simulink model "Solar_Seguidor_V2"  (R2021b)
settings: Solver=ode1  StartTime=0.0  StopTime=10  FixedStep=25e-6  RelTol=1e-3
PostLoadFcn:
  | %clc; clear all; close all;
  | %%%%%%%%%%%%%%%%%%%%%%%%%%%%%%%%%%%%%%%%%%%%%%%%
  | %%%%%%%%% Solar seguidor de rede %%%%%%%%%%
  | %%%%%%%%%%%%%%%%%%%%%%%%%%%%%%%%%%%%%%%%%%%%%%%%
  | %%%% Nominal Parameters %%%%
  | Pnom = 16e3;                                         % Potencia Nominal
  | Vnom_rms = 210;                                    % V linha rms
  | Vnom_peak = sqrt(2/3)*Vnom_rms;                     % V fase pico
  | FP_min = 1;                                       % Para suporte de reativo
  | Snom = Pnom/FP_min;                                 % Potencia aparente
  | Irms = Pnom/(sqrt(3)*Vnom_rms);                     % Ig rms
  | Inom_peak = Irms*sqrt(2);                           % Ig pico
  | Zbase = Vnom_peak/Inom_peak;                        % Impedancia Base
  | f = 60;                                             % Freq nominal
  | wnom = 2*pi*60;                                     % Freq Ang. nominal
  | m = 0.805;                                            % Indice mod nominal
  | Vdc = 2*(Vnom_peak/m);                              % Vcc
  | Vdc_2 = Vdc/2;                                      % Metade Vcc
  | Kconv = Zbase;                                      % Ganho conversor
  | %%%% Transformer %%%%
  | S_trafo = 250e3;                                      % transformer apparent power
  | Vrms_high = 400;                                   % transformer secondary voltage - Wye connection
  | Vrms_low = 210;                                   % transformer primary voltage - Delta connection
  | N = Vrms_high/Vrms_low;                             % transformation relationship
  | X_pu_trafo = 0.03;                                 % transformer p.u. reactance
  | Zb_trafo_high = ((Vrms_high)^2)/S_trafo;            % secondary base impedance
  | Zb_trafo = ((Vnom_rms)^2)/S_trafo;                  % primary base impedance
  | L_trafo = (X_pu_trafo*Zb_trafo)/wnom;               % primary inductance
  | %%%% LCL Filter Project %%%%
  | fsw = 105*60;%105*60;                                         % switching frequency
  | ripple = 0.05;                                       % current ripple
  | L1 = Vdc/(6*ripple*Inom_peak*fsw);                  % inductor L1
  |  RL1 = 0.005;                                        % L1 resistance
  |  Cbase = 1/(wnom*Kconv);                             % base capacitance
  |  Cf = 0.05*Cbase;                                    % filter capacitor
  | % Calculo do filtro
  | Sbase = 16e3;
  | %Sbase = 200e3*1.12;
  | V_LL = 210;
  | V_LG = 210/sqrt(3);
  | Vbase = V_LG*sqrt(2);
  | Ibase = (Sbase*sqrt(2))/(V_LG*3)*sqrt(3/2);
  | Zbase = (V_LL^2)/Sbase;
  | Rbase = Zbase;
  | Xbase = Zbase;
  | Lbase = Xbase/(2*pi*60);
  | Cbase = 1/(Xbase*2*pi*60);
  | w = 2*pi*60;
  | Q = 70;
  | Lf = 0.15*Lbase;
  | Cf = 0.05*Cbase;
  | fc = 1/(2*pi*sqrt(Lf*Cf));
  | R = (w*Lf)/Q;
  | Lf = L1;
  | R = RL1;
  | ka=0.2;                                             % attenuation factor
  | L2 = (sqrt(1/(ka^2))+1)/(Cf*((2*pi*fsw)^2));        % inductor L2
  | RL2 = 0.005;                                        % L2 resistance
  | w_res = sqrt((L1+L2+L_trafo)/(L1*L2*Cf));           % resonant angular frequency
  | f_res = w_res/(2*pi);                               % resonant frequency
  | ... (+31 lines)
InitFcn:
  | %clc; clear all; close all;
  | %%%%%%%%%%%%%%%%%%%%%%%%%%%%%%%%%%%%%%%%%%%%%%%%
  | %%%%%%%%% Solar seguidor de rede %%%%%%%%%%
  | %%%%%%%%%%%%%%%%%%%%%%%%%%%%%%%%%%%%%%%%%%%%%%%%
  | %%%% Nominal Parameters %%%%
  | Pnom = 16e3;                                         % Potencia Nominal
  | Vnom_rms = 210;                                    % V linha rms
  | Vnom_peak = sqrt(2/3)*Vnom_rms;                     % V fase pico
  | FP_min = 1;                                       % Para suporte de reativo
  | Snom = Pnom/FP_min;                                 % Potencia aparente
  | Irms = Pnom/(sqrt(3)*Vnom_rms);                     % Ig rms
  | Inom_peak = Irms*sqrt(2);                           % Ig pico
  | Zbase = Vnom_peak/Inom_peak;                        % Impedancia Base
  | f = 60;                                             % Freq nominal
  | wnom = 2*pi*60;                                     % Freq Ang. nominal
  | m = 0.805;                                            % Indice mod nominal
  | Vdc = 2*(Vnom_peak/m);                              % Vcc
  | Vdc_2 = Vdc/2;                                      % Metade Vcc
  | Kconv = Zbase;                                      % Ganho conversor
  | %%%% Transformer %%%%
  | S_trafo = 250e3;                                      % transformer apparent power
  | Vrms_high = 400;                                   % transformer secondary voltage - Wye connection
  | Vrms_low = 210;                                   % transformer primary voltage - Delta connection
  | N = Vrms_high/Vrms_low;                             % transformation relationship
  | X_pu_trafo = 0.03;                                 % transformer p.u. reactance
  | Zb_trafo_high = ((Vrms_high)^2)/S_trafo;            % secondary base impedance
  | Zb_trafo = ((Vnom_rms)^2)/S_trafo;                  % primary base impedance
  | L_trafo = (X_pu_trafo*Zb_trafo)/wnom;               % primary inductance
  | %%%% LCL Filter Project %%%%
  | fsw = 105*60;%105*60;                                         % switching frequency
  | ripple = 0.05;                                       % current ripple
  | L1 = Vdc/(6*ripple*Inom_peak*fsw);                  % inductor L1
  |  RL1 = 0.005;                                        % L1 resistance
  |  Cbase = 1/(wnom*Kconv);                             % base capacitance
  |  Cf = 0.05*Cbase;                                    % filter capacitor
  | % Calculo do filtro
  | Sbase = 16e3;
  | %Sbase = 200e3*1.12;
  | V_LL = 210;
  | V_LG = 210/sqrt(3);
  | Vbase = V_LG*sqrt(2);
  | Ibase = (Sbase*sqrt(2))/(V_LG*3)*sqrt(3/2);
  | Zbase = (V_LL^2)/Sbase;
  | Rbase = Zbase;
  | Xbase = Zbase;
  | Lbase = Xbase/(2*pi*60);
  | Cbase = 1/(Xbase*2*pi*60);
  | w = 2*pi*60;
  | Q = 70;
  | Lf = 0.15*Lbase;
  | Cf = 0.05*Cbase;
  | fc = 1/(2*pi*sqrt(Lf*Cf));
  | R = (w*Lf)/Q;
  | Lf = L1;
  | R = RL1;
  | ka=0.2;                                             % attenuation factor
  | L2 = (sqrt(1/(ka^2))+1)/(Cf*((2*pi*fsw)^2));        % inductor L2
  | RL2 = 0.005;                                        % L2 resistance
  | w_res = sqrt((L1+L2+L_trafo)/(L1*L2*Cf));           % resonant angular frequency
  | f_res = w_res/(2*pi);                               % resonant frequency
  | ... (+31 lines)
undefined symbols (not defined in the file): D1, Delta, DERS_models, DiscIntNeverNeededParam, eHS, I, Ia_PV, Ib_PV, Ic_PV, Left, parameter_set_id, ph, PV_system, type, V, Va_grid, Vb_grid, Vc_grid
libraries: powerlib_meascontrol x17, rtlab x14, spsThreePhaseSeriesRLCBranchLib x9, spsCurrentMeasurementLib x9, artemis x7, spsThreePhaseVIMeasurementLib x6, slpidlib x6, rteventslib x6, spsabctodq0Lib x4, spsThreePhaseTransformerTwoWindingsLib x3, simulink x3, spsPVArrayLib x3
(part 2 of 4)

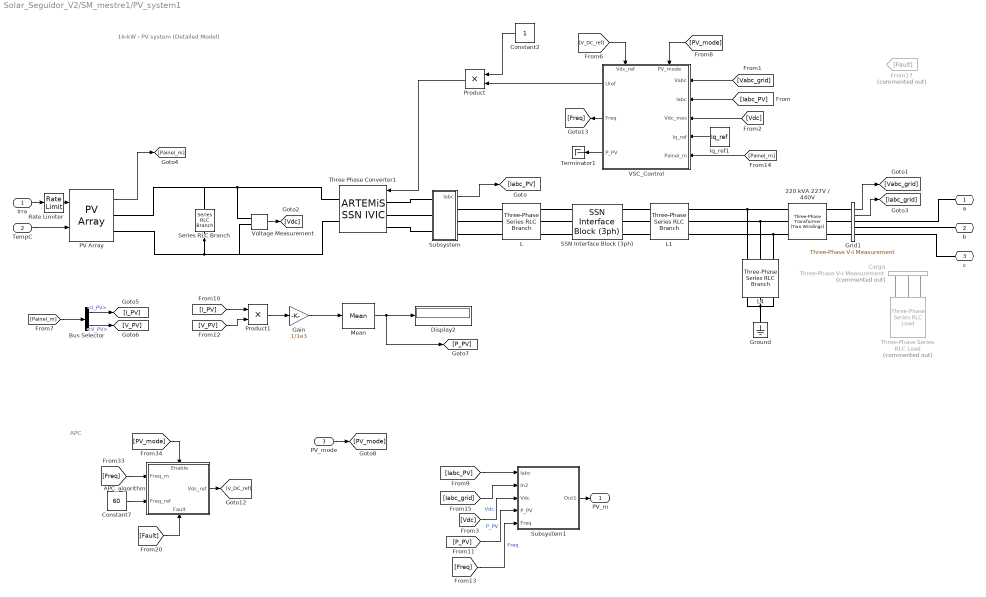
== system Solar_Seguidor_V2/SM_mestre1/PV_system1 ==
  note: APC
  note: 16-kW - PV system (Detailed Model)
  Irra : Inport
  TempC : Inport  Port=2
  PV_mode : Inport  Port=3
  220 kVA 227V / 440V : spsThreePhaseTransformerTwoWindingsLib/Three-Phase Transformer (Two Windings)  Winding1Connection=Yg  Winding2Connection=Delta (D1)  CoreType=Three single-phase transformers  SetSaturation=off  Hysteresis=off  DataFile='hysteresis'  SetInitialFlux=off  Measurements=None  UNITS=pu  NominalPower=[220e3 , 60 ]  Winding1=[400 , 0.001 , 0.03 ]  Winding2=[210 , 0.001 , 0.03 ]  Rm=500  Lm=500  L0=0.5  Saturation=[ 0,0 ; 0.0024,1.2 ; 1.0,1.52 ]  InitialFluxes=[ 0.8 , -0.8 , 0.7 ]  BreakLoop=off  DiscreteSolver=Trapezoidal iterative  DataType=off  TransfoNumber=0
  APC_algorithm : Subsystem
      settings: PortSchema="{\"entries\":[{\"content\":{\"sides\":[{\"content\":{\"connectorIds\":[\"In1\",\"In2\"]},\"type\":\"ConnectorPlacement.EquallySpacedRectSide\",\"uuid\":\"40656380-5e11-4201-a16e-0974ed2bdfa3\"},{\"content\":{\"connectorIds\":[\"Out1\"],\"side\":\"RIGHT\"},\"type\":\"ConnectorPlacement.EquallySpacedRectSide\",\"uuid\":\"b720f4a2-445d-4911-b95b-a16e7ba2ef90\"},{\"content\":{\"connectorIds\":[\"In3\"],\"side\":\"TOP\"},\"type\":\"ConnectorPlacement.EquallySpacedRectSide\",\"uuid\":\"61735eee-8c6f-4b86-833d-6912c6cea25a\"},{\"content\":{\"connectorIds\":[\"In4\"],\"side\":\"BOTTOM\"},\"type\":\"ConnectorPlacement.EquallySpacedRectSide\",\"uuid\":\"0dbf41d0-9732-4713-8148-d584ab86d8ba\"},{\"content\":{\"connectorIds\":[],\"side\":\"HIDDEN\"},\"type\":\"ConnectorPlacement.EquallySpacedRectSide\",\"uuid\":\"d2c68c6b-be31-4766-a941-11238d66741c\"}]},\"type\":\"ConnectorPlacement.EquallySpacedConnector\",\"uuid\":\"e0287d46-a6c7-46a5-bd63-f4e94fb98690\"}],\"packageUris\":[\"http://schema.mathworks.com/mf0/Connector/R2020b\"],\"version\":\"1.0\"}"
  Bus Selector : BusSelector  OutputSignals=I_PV,V_PV
  Carga : spsThreePhaseVIMeasurementLib/Three-Phase V-I Measurement  Commented=on  VoltageMeasurement=phase-to-ground  SetLabelV=on  LabelV=Vcarga  Vpu=off  VpuLL=off  CurrentMeasurement=yes  SetLabelI=on  LabelI=Icarga  Ipu=off  Pbase=100e6  Vbase=500e3  OutputType=Magnitude  PhasorSimulation=off  PSBequivalent=0
  Constant2 : Constant
  Constant7 : Constant  Value=60
  Display2 : Display
  From17 : From  Commented=on  GotoTag=Fault
  Gain : Gain  Gain=1/1e3
  Grid1 : spsThreePhaseVIMeasurementLib/Three-Phase V-I Measurement  VoltageMeasurement=phase-to-ground  SetLabelV=off  LabelV=Vabc_grid  Vpu=off  VpuLL=off  CurrentMeasurement=yes  SetLabelI=off  LabelI=Iabc_grid  Ipu=off  Pbase=100e6  Vbase=500e3  OutputType=Magnitude  PhasorSimulation=off  PSBequivalent=0
  Ground : spsGroundLib/Ground  LConnTagsString=a
  Iq_ref1 : Constant  Value=Iq_ref
  L : spsThreePhaseSeriesRLCBranchLib/Three-Phase Series RLC Branch  LConnTagsString=A|B|C  RConnTagsString=A|B|C  BranchType=R  Resistance=R  Inductance=500e-6/2  Capacitance=inf  Measurements=None
  L1 : spsThreePhaseSeriesRLCBranchLib/Three-Phase Series RLC Branch  LConnTagsString=A|B|C  RConnTagsString=A|B|C  BranchType=L  Resistance=500e-6*377/50/2  Inductance=Lf  Capacitance=inf  Measurements=None
  L4 : spsThreePhaseSeriesRLCBranchLib/Three-Phase Series RLC Branch  LConnTagsString=A|B|C  RConnTagsString=A|B|C  BranchType=R  Resistance=1e8  Inductance=Lf  Capacitance=Cf  Measurements=None
  Mean : spsMeanLib/Mean  Freq=60  Vinit=0  Ts=0
  PV Array : spsPVArrayLib/PV Array  Npar=5  Nser=14  PlotType=array @ 1000 W/m2 & specified temperatures  S_vec=[ 1000]  Temp_C_vec=[ 25 ]  ModuleName=Trina Solar TSM-240PA05.30  PlotWhenSelected=off  Pm=239.856  Ncell=60  Voc=37.2  Isc=8.37  Vm=30.4  Im=7.89  beta_Voc_pc=-0.35  alpha_Isc_pc=0.06  beta_Voc=-0.1302  alpha_Isc=0.005022  IL=8.3942  I0=1.9964e-10  nI=0.98701  Rsh=355.1808  Rs=0.28785  RobustModel=off  RobustCellTemperature=313.3991  BAL=on  Tc=1e-6  Tfilter=5e-5
      settings: AttributesFormatString=|
      | %<ModuleName>
      | %<Nser>-module string
      | %<Npar> parallel strings
  Product : Product
  Product1 : Product
  Rate Limiter : RateLimiter  RisingSlewLimit=5000  FallingSlewLimit=-5000  SampleTimeMode=inherited  LinearizeAsGain=off
  SSN Interface Block (3ph) : artemis/SSN/Nodal Interface Blocks/SSN Interface Block (3ph)  nb_phase=3  nb_port=2  p1_type=I-type(Left)  p2_type=V-type (Right)  p3_type=V-type(Left)  p4_type=V-type(Left)  p5_type=V-type(Left)  p6_type=V-type(Left)  p7_type=V-type(Left)  p8_type=V-type(Left)  p9_type=V-type(Left)  p10_type=V-type(Left)  p11_type=V-type(Left)  p12_type=V-type(Left)  p13_type=V-type(Left)  p14_type=V-type(Left)  p15_type=V-type(Left)  p16_type=V-type(Left)  I_port_shunt_resistance=1e9
  Series RLC Branch : spsSeriesRLCBranchLib/Series RLC Branch  LConnTagsString=__new0  RConnTagsString=__new0  BranchType=C  Resistance=1  Inductance=1e-3  SetiL0=off  InitialCurrent=0  Capacitance=C_cc_proj  Setx0=on  InitialVoltage=Vdc  Measurements=None
  Subsystem : Subsystem
  Subsystem1 : Subsystem
  Terminator1 : Terminator
  Three Phase Converter1 : ssn_inverter_model/ARTEMiS SSN IVIC  Arms=3  SnubberResistance=800  SnubberCapacitance=inf  Device=IGBT / Diodes  Ron=Ron  Lon=0  ForwardVoltages=[0.001 0.001]  ForwardVoltage=0  GTOparameters=[ 10e-6 , 20e-6 ]  IGBTparameters=[ 1e-6 , 2e-6 ]*0  Measurements=None  Measurements_2=None  converterType=Rectifier
  Three-Phase Series RLC Load : spsThreePhaseSeriesRLCLoadLib/Three-Phase Series RLC Load  Commented=on  LConnTagsString=A|B|C  Configuration=Y (grounded)  NominalVoltage=227  Vabc=[1e3 1e3 1e3]  Vabcp=[1e3 1e3 1e3]  NominalFrequency=60  UnbalancedPower=off  ActivePower=80e3  InductivePower=15e3  CapacitivePower=0  Pabc=[10e3 9e3 11e3]  QLabc=[100 90 110]  QCabc=[100 90 110]  Pabcp=[10e3 9e3 11e3]  QLabcp=[100 90 110]  QCabcp=[100 90 110]  Measurements=None  LoadType=constant Z
  VSC_Control : Subsystem
      settings: PortSchema="{\"entries\":[{\"content\":{\"sides\":[{\"content\":{\"connectorIds\":[\"In1\",\"In2\",\"In3\",\"In4\",\"In5\"]},\"type\":\"ConnectorPlacement.EquallySpacedRectSide\",\"uuid\":\"45e52e2a-5d2e-4b01-a357-9d3073978641\"},{\"content\":{\"connectorIds\":[\"Out1\",\"Out2\",\"Out3\"],\"side\":\"RIGHT\"},\"type\":\"ConnectorPlacement.EquallySpacedRectSide\",\"uuid\":\"500a659a-c60e-4c3f-b5c2-04d8fe26286a\"},{\"content\":{\"connectorIds\":[\"In6\",\"In7\"],\"side\":\"TOP\"},\"type\":\"ConnectorPlacement.EquallySpacedRectSide\",\"uuid\":\"e5a9e837-077a-4c9c-b808-725d6018483b\"},{\"content\":{\"connectorIds\":[],\"side\":\"HIDDEN\"},\"type\":\"ConnectorPlacement.EquallySpacedRectSide\",\"uuid\":\"1c877ae8-e0c9-4faf-8b8c-99cd40b797b6\"}]},\"type\":\"ConnectorPlacement.EquallySpacedConnector\",\"uuid\":\"17a691b0-ccba-4cde-88e8-165a3a0c6333\"}],\"packageUris\":[\"http://schema.mathworks.com/mf0/Connector/R2020b\"],\"version\":\"1.0\"}"
  Voltage Measurement : spsVoltageMeasurementLib/Voltage Measurement  PhasorSimulation=off  OutputType=Complex  PSBequivalent=0
  a : PMIOPort  Side=Right
  b : PMIOPort  Port=2  Side=Right
  c : PMIOPort  Port=3  Side=Right
  PV_m : Outport
  wires:
  Subsystem1/1(Out1) -> PV_m/1
  [Freq] -> Subsystem1/5(Freq)  "Freq"
  [P_PV] -> Subsystem1/4(P_PV)  "P_PV"
  [Vdc] -> Subsystem1/3(Vdc)  "Vdc"
  [Iabc_grid] -> Subsystem1/2(In2)
  [Iabc_PV] -> Subsystem1/1(Iabc)
  PV_mode/1 -> [PV_mode]
  Grid1/2 -> [Iabc_grid]
  [Painel_m] -> VSC_Control/5(Painel_m)
  TempC/1 -> PV Array/2
  Irra/1 -> Rate Limiter/1
  Bus Selector/2 -> [V_PV]  "<V_PV>"
  VSC_Control/3(P_PV) -> Terminator1/1
  Mean/1 -> Display2/1, [P_PV]
  Constant7/1 -> APC_algorithm/2(Freq_ref)
  [Fault] -> APC_algorithm/4(Fault)
  APC_algorithm/1(Vdc_ref) -> [V_DC_ref]
  [Painel_m] -> Bus Selector/1
  Grid1/1 -> [Vabc_grid]
  [Vdc] -> VSC_Control/3(Vdc_mes)
  Product/1 -> Three Phase Converter1/1
  Voltage Measurement/1 -> [Vdc]
  [Vabc_grid] -> VSC_Control/1(Vabc)
  [PV_mode] -> VSC_Control/6(PV_mode)
  Bus Selector/1 -> [I_PV]  "<I_PV>"
  Gain/1 -> Mean/1
  [Iabc_PV] -> VSC_Control/2(Iabc)
  Iq_ref1/1 -> VSC_Control/4(Iq_ref)
  Rate Limiter/1 -> PV Array/1
  VSC_Control/2(Freq) -> [Freq]
  [V_DC_ref] -> VSC_Control/7(Vdc_ref)
  [V_PV] -> Product1/2
  Product1/1 -> Gain/1
  VSC_Control/1(Uref) -> Product/2
  [PV_mode] -> APC_algorithm/3(Enable)
  [Freq] -> APC_algorithm/1(Freq_m)
  Constant2/1 -> Product/1
  Subsystem/1(Iabc) -> [Iabc_PV]
  PV Array/1 -> [Painel_m]
  [I_PV] -> Product1/1
  connections:
  c/RConn1 -- Grid1/RConn3
  b/RConn1 -- Grid1/RConn2
  Grid1/LConn3 -- 220 kVA 227V / 440V/LConn3
  Grid1/LConn1 -- 220 kVA 227V / 440V/LConn1
  L1/LConn2 -- SSN Interface Block (3ph)/RConn2
  Carga/RConn3 -- Three-Phase Series RLC Load/LConn1
  Subsystem/RConn3 -- L/LConn3
  SSN Interface Block (3ph)/LConn3 -- L/RConn3
  Three Phase Converter1/LConn2 -- Subsystem/LConn2
  Subsystem/LConn3 -- Three Phase Converter1/LConn3
  Subsystem/RConn2 -- L/LConn2
  Grid1/LConn2 -- 220 kVA 227V / 440V/LConn2
  Series RLC Branch/RConn1 -- PV Array/RConn2 -- Three Phase Converter1/RConn2 -- Voltage Measurement/LConn2
  Carga/RConn2 -- Three-Phase Series RLC Load/LConn2
  L4/LConn1 -- 220 kVA 227V / 440V/RConn1 -- L1/RConn1
  Subsystem/LConn1 -- Three Phase Converter1/LConn1
  SSN Interface Block (3ph)/LConn2 -- L/RConn2
  220 kVA 227V / 440V/RConn2 -- L4/LConn2 -- L1/RConn2
  220 kVA 227V / 440V/RConn3 -- L4/LConn3 -- L1/RConn3
  Voltage Measurement/LConn1 -- PV Array/RConn1 -- Series RLC Branch/LConn1 -- Three Phase Converter1/RConn1
  L1/LConn1 -- SSN Interface Block (3ph)/RConn1
  Carga/RConn1 -- Three-Phase Series RLC Load/LConn3
  a/RConn1 -- Grid1/RConn1
  L4/RConn2 -- Ground/LConn1 -- L4/RConn3 -- L4/RConn1
  L/RConn1 -- SSN Interface Block (3ph)/LConn1
  L1/LConn3 -- SSN Interface Block (3ph)/RConn3
  Subsystem/RConn1 -- L/LConn1

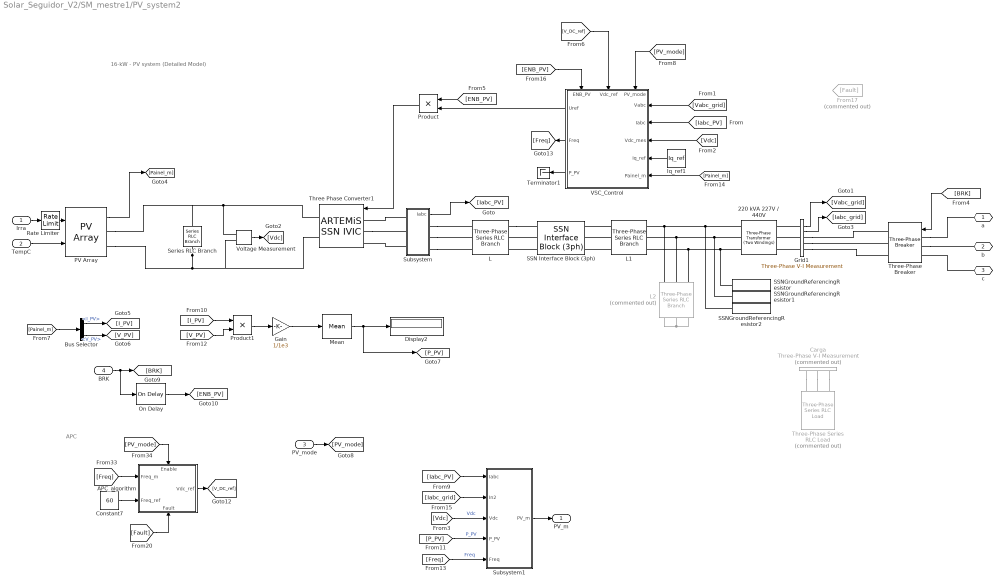
== system Solar_Seguidor_V2/SM_mestre1/PV_system2 ==
  note: APC
  note: 16-kW - PV system (Detailed Model)
  Irra : Inport
  TempC : Inport  Port=2
  PV_mode : Inport  Port=3
  BRK : Inport  Port=4
  220 kVA 227V / 440V : spsThreePhaseTransformerTwoWindingsLib/Three-Phase Transformer (Two Windings)  Winding1Connection=Yg  Winding2Connection=Delta (D1)  CoreType=Three single-phase transformers  SetSaturation=off  Hysteresis=off  DataFile='hysteresis'  SetInitialFlux=off  Measurements=None  UNITS=pu  NominalPower=[220e3 , 60 ]  Winding1=[400 , 0.001 , 0.03 ]  Winding2=[210 , 0.001 , 0.03 ]  Rm=500  Lm=500  L0=0.5  Saturation=[ 0,0 ; 0.0024,1.2 ; 1.0,1.52 ]  InitialFluxes=[ 0.8 , -0.8 , 0.7 ]  BreakLoop=off  DiscreteSolver=Trapezoidal iterative  DataType=off  TransfoNumber=0
  APC_algorithm : Subsystem
      settings: PortSchema="{\"entries\":[{\"content\":{\"sides\":[{\"content\":{\"connectorIds\":[\"In1\",\"In2\"]},\"type\":\"ConnectorPlacement.EquallySpacedRectSide\",\"uuid\":\"40656380-5e11-4201-a16e-0974ed2bdfa3\"},{\"content\":{\"connectorIds\":[\"Out1\"],\"side\":\"RIGHT\"},\"type\":\"ConnectorPlacement.EquallySpacedRectSide\",\"uuid\":\"b720f4a2-445d-4911-b95b-a16e7ba2ef90\"},{\"content\":{\"connectorIds\":[\"In3\"],\"side\":\"TOP\"},\"type\":\"ConnectorPlacement.EquallySpacedRectSide\",\"uuid\":\"61735eee-8c6f-4b86-833d-6912c6cea25a\"},{\"content\":{\"connectorIds\":[\"In4\"],\"side\":\"BOTTOM\"},\"type\":\"ConnectorPlacement.EquallySpacedRectSide\",\"uuid\":\"0dbf41d0-9732-4713-8148-d584ab86d8ba\"},{\"content\":{\"connectorIds\":[],\"side\":\"HIDDEN\"},\"type\":\"ConnectorPlacement.EquallySpacedRectSide\",\"uuid\":\"d2c68c6b-be31-4766-a941-11238d66741c\"}]},\"type\":\"ConnectorPlacement.EquallySpacedConnector\",\"uuid\":\"e0287d46-a6c7-46a5-bd63-f4e94fb98690\"}],\"packageUris\":[\"http://schema.mathworks.com/mf0/Connector/R2020b\"],\"version\":\"1.0\"}"
  Bus Selector : BusSelector  OutputSignals=I_PV,V_PV
  Carga : spsThreePhaseVIMeasurementLib/Three-Phase V-I Measurement  Commented=on  VoltageMeasurement=phase-to-ground  SetLabelV=on  LabelV=Vcarga  Vpu=off  VpuLL=off  CurrentMeasurement=yes  SetLabelI=on  LabelI=Icarga  Ipu=off  Pbase=100e6  Vbase=500e3  OutputType=Magnitude  PhasorSimulation=off  PSBequivalent=0
  Constant7 : Constant  Value=60
  Display2 : Display
  From17 : From  Commented=on  GotoTag=Fault
  Gain : Gain  Gain=1/1e3
  Grid1 : spsThreePhaseVIMeasurementLib/Three-Phase V-I Measurement  VoltageMeasurement=phase-to-ground  SetLabelV=off  LabelV=Vabc_grid  Vpu=off  VpuLL=off  CurrentMeasurement=yes  SetLabelI=off  LabelI=Iabc_grid  Ipu=off  Pbase=100e6  Vbase=500e3  OutputType=Magnitude  PhasorSimulation=off  PSBequivalent=0
  Iq_ref1 : Constant  Value=Iq_ref
  L : spsThreePhaseSeriesRLCBranchLib/Three-Phase Series RLC Branch  LConnTagsString=A|B|C  RConnTagsString=A|B|C  BranchType=R  Resistance=R  Inductance=500e-6/2  Capacitance=inf  Measurements=None
  L1 : spsThreePhaseSeriesRLCBranchLib/Three-Phase Series RLC Branch  LConnTagsString=A|B|C  RConnTagsString=A|B|C  BranchType=L  Resistance=500e-6*377/50/2  Inductance=Lf  Capacitance=inf  Measurements=None
  L2 : spsThreePhaseSeriesRLCBranchLib/Three-Phase Series RLC Branch  Commented=on  LConnTagsString=A|B|C  RConnTagsString=A|B|C  BranchType=RC  Resistance=Cf*377/50/2  Inductance=Lf  Capacitance=Cf  Measurements=None
  Mean : spsMeanLib/Mean  Freq=60  Vinit=0  Ts=0
  On Delay : spsOnDelayLib/On Delay  DelayType=On delay  delay=0.25  ic=1  Ts=Ts
      settings: SourceProductBaseCode=PS
  PV Array : spsPVArrayLib/PV Array  Npar=5  Nser=14  PlotType=array @ 1000 W/m2 & specified temperatures  S_vec=[ 1000]  Temp_C_vec=[ 25 ]  ModuleName=Trina Solar TSM-240PA05.30  PlotWhenSelected=off  Pm=239.856  Ncell=60  Voc=37.2  Isc=8.37  Vm=30.4  Im=7.89  beta_Voc_pc=-0.35  alpha_Isc_pc=0.06  beta_Voc=-0.1302  alpha_Isc=0.005022  IL=8.3942  I0=1.9964e-10  nI=0.98701  Rsh=355.1808  Rs=0.28785  RobustModel=off  RobustCellTemperature=313.3991  BAL=on  Tc=1e-6  Tfilter=5e-5
      settings: AttributesFormatString=|
      | %<ModuleName>
      | %<Nser>-module string
      | %<Npar> parallel strings
  Product : Product
  Product1 : Product
  Rate Limiter : RateLimiter  RisingSlewLimit=5000  FallingSlewLimit=-5000  SampleTimeMode=inherited  LinearizeAsGain=off
  SSN Interface Block (3ph) : artemis/SSN/Nodal Interface Blocks/SSN Interface Block (3ph)  nb_phase=3  nb_port=2  p1_type=I-type(Left)  p2_type=V-type (Right)  p3_type=V-type(Left)  p4_type=V-type(Left)  p5_type=V-type(Left)  p6_type=V-type(Left)  p7_type=V-type(Left)  p8_type=V-type(Left)  p9_type=V-type(Left)  p10_type=V-type(Left)  p11_type=V-type(Left)  p12_type=V-type(Left)  p13_type=V-type(Left)  p14_type=V-type(Left)  p15_type=V-type(Left)  p16_type=V-type(Left)  I_port_shunt_resistance=1e9
  SSNGroundReferencingResistor : artemis/SSN/SSNGroundReferencingResistor  Rr=1e8
  SSNGroundReferencingResistor1 : artemis/SSN/SSNGroundReferencingResistor  Rr=1e8
  SSNGroundReferencingResistor2 : artemis/SSN/SSNGroundReferencingResistor  Rr=1e8
  Series RLC Branch : spsSeriesRLCBranchLib/Series RLC Branch  LConnTagsString=__new0  RConnTagsString=__new0  BranchType=C  Resistance=1  Inductance=1e-3  SetiL0=off  InitialCurrent=0  Capacitance=C_cc_proj  Setx0=on  InitialVoltage=Vdc  Measurements=None
  Subsystem : Subsystem
  Subsystem1 : Subsystem
  Terminator1 : Terminator
  Three Phase Converter1 : ssn_inverter_model/ARTEMiS SSN IVIC  Arms=3  SnubberResistance=800  SnubberCapacitance=inf  Device=IGBT / Diodes  Ron=Ron  Lon=0  ForwardVoltages=[0.001 0.001]  ForwardVoltage=0  GTOparameters=[ 10e-6 , 20e-6 ]  IGBTparameters=[ 1e-6 , 2e-6 ]*0  Measurements=None  Measurements_2=None  converterType=Rectifier
  Three-Phase Series RLC Load : spsThreePhaseSeriesRLCLoadLib/Three-Phase Series RLC Load  Commented=on  LConnTagsString=A|B|C  Configuration=Y (grounded)  NominalVoltage=227  Vabc=[1e3 1e3 1e3]  Vabcp=[1e3 1e3 1e3]  NominalFrequency=60  UnbalancedPower=off  ActivePower=80e3  InductivePower=15e3  CapacitivePower=0  Pabc=[10e3 9e3 11e3]  QLabc=[100 90 110]  QCabc=[100 90 110]  Pabcp=[10e3 9e3 11e3]  QLabcp=[100 90 110]  QCabcp=[100 90 110]  Measurements=None  LoadType=constant Z
  Three-Phase Breaker : spsThreePhaseBreakerLib/Three-Phase Breaker  InitialState=open  SwitchA=on  SwitchB=on  SwitchC=on  SwitchTimes="[1/60  5/60]"  External=on  BreakerResistance=0.01  SnubberResistance=1e6  SnubberCapacitance=inf  Measurements=None
  VSC_Control : Subsystem
      settings: PortSchema="{\"entries\":[{\"content\":{\"sides\":[{\"content\":{\"connectorIds\":[\"In1\",\"In2\",\"In3\",\"In4\",\"In5\"]},\"type\":\"ConnectorPlacement.EquallySpacedRectSide\",\"uuid\":\"45e52e2a-5d2e-4b01-a357-9d3073978641\"},{\"content\":{\"connectorIds\":[\"Out1\",\"Out2\",\"Out3\"],\"side\":\"RIGHT\"},\"type\":\"ConnectorPlacement.EquallySpacedRectSide\",\"uuid\":\"500a659a-c60e-4c3f-b5c2-04d8fe26286a\"},{\"content\":{\"connectorIds\":[\"In6\",\"In7\",\"In8\"],\"side\":\"TOP\"},\"type\":\"ConnectorPlacement.EquallySpacedRectSide\",\"uuid\":\"e5a9e837-077a-4c9c-b808-725d6018483b\"},{\"content\":{\"connectorIds\":[],\"side\":\"HIDDEN\"},\"type\":\"ConnectorPlacement.EquallySpacedRectSide\",\"uuid\":\"1c877ae8-e0c9-4faf-8b8c-99cd40b797b6\"}]},\"type\":\"ConnectorPlacement.EquallySpacedConnector\",\"uuid\":\"17a691b0-ccba-4cde-88e8-165a3a0c6333\"}],\"packageUris\":[\"http://schema.mathworks.com/mf0/Connector/R2020b\"],\"version\":\"1.0\"}"
  Voltage Measurement : spsVoltageMeasurementLib/Voltage Measurement  PhasorSimulation=off  OutputType=Complex  PSBequivalent=0
  a : PMIOPort  Side=Right
  b : PMIOPort  Port=2  Side=Right
  c : PMIOPort  Port=3  Side=Right
  PV_m : Outport
  wires:
  Subsystem1/1(PV_m) -> PV_m/1
  [Freq] -> Subsystem1/5(Freq)  "Freq"
  [P_PV] -> Subsystem1/4(P_PV)  "P_PV"
  [Vdc] -> Subsystem1/3(Vdc)  "Vdc"
  [Iabc_grid] -> Subsystem1/2(In2)
  [Iabc_PV] -> Subsystem1/1(Iabc)
  PV_mode/1 -> [PV_mode]
  Grid1/2 -> [Iabc_grid]
  [Painel_m] -> VSC_Control/5(Painel_m)
  TempC/1 -> PV Array/2
  Irra/1 -> Rate Limiter/1
  Bus Selector/2 -> [V_PV]  "<V_PV>"
  VSC_Control/3(P_PV) -> Terminator1/1
  Mean/1 -> Display2/1, [P_PV]
  Constant7/1 -> APC_algorithm/2(Freq_ref)
  [Fault] -> APC_algorithm/4(Fault)
  APC_algorithm/1(Vdc_ref) -> [V_DC_ref]
  [Painel_m] -> Bus Selector/1
  Grid1/1 -> [Vabc_grid]
  [Vdc] -> VSC_Control/3(Vdc_mes)
  Product/1 -> Three Phase Converter1/1
  Voltage Measurement/1 -> [Vdc]
  [Vabc_grid] -> VSC_Control/1(Vabc)
  [PV_mode] -> VSC_Control/6(PV_mode)
  Bus Selector/1 -> [I_PV]  "<I_PV>"
  Gain/1 -> Mean/1
  [Iabc_PV] -> VSC_Control/2(Iabc)
  Iq_ref1/1 -> VSC_Control/4(Iq_ref)
  Rate Limiter/1 -> PV Array/1
  VSC_Control/2(Freq) -> [Freq]
  [V_DC_ref] -> VSC_Control/7(Vdc_ref)
  [V_PV] -> Product1/2
  Product1/1 -> Gain/1
  VSC_Control/1(Uref) -> Product/2
  [PV_mode] -> APC_algorithm/3(Enable)
  [Freq] -> APC_algorithm/1(Freq_m)
  Subsystem/1(Iabc) -> [Iabc_PV]
  PV Array/1 -> [Painel_m]
  [I_PV] -> Product1/1
  [BRK] -> Three-Phase Breaker/1
  BRK/1 -> On Delay/1, [BRK]
  On Delay/1 -> [ENB_PV]
  [ENB_PV] -> Product/1
  [ENB_PV] -> VSC_Control/8(ENB_PV)
  connections:
  Grid1/LConn3 -- 220 kVA 227V / 440V/LConn3
  Grid1/LConn1 -- 220 kVA 227V / 440V/LConn1
  L1/LConn2 -- SSN Interface Block (3ph)/RConn2
  Carga/RConn3 -- Three-Phase Series RLC Load/LConn1
  Subsystem/RConn3 -- L/LConn3
  SSN Interface Block (3ph)/LConn3 -- L/RConn3
  Three Phase Converter1/LConn2 -- Subsystem/LConn2
  Subsystem/LConn3 -- Three Phase Converter1/LConn3
  Subsystem/RConn2 -- L/LConn2
  Grid1/LConn2 -- 220 kVA 227V / 440V/LConn2
  Series RLC Branch/RConn1 -- PV Array/RConn2 -- Three Phase Converter1/RConn2 -- Voltage Measurement/LConn2
  Carga/RConn2 -- Three-Phase Series RLC Load/LConn2
  220 kVA 227V / 440V/RConn1 -- SSNGroundReferencingResistor2/RConn1 -- L2/LConn1 -- L1/RConn1
  Subsystem/LConn1 -- Three Phase Converter1/LConn1
  SSN Interface Block (3ph)/LConn2 -- L/RConn2
  220 kVA 227V / 440V/RConn2 -- SSNGroundReferencingResistor1/RConn1 -- L2/LConn2 -- L1/RConn2
  220 kVA 227V / 440V/RConn3 -- SSNGroundReferencingResistor/RConn1 -- L2/LConn3 -- L1/RConn3
  Voltage Measurement/LConn1 -- PV Array/RConn1 -- Series RLC Branch/LConn1 -- Three Phase Converter1/RConn1
  L1/LConn1 -- SSN Interface Block (3ph)/RConn1
  Carga/RConn1 -- Three-Phase Series RLC Load/LConn3
  L/RConn1 -- SSN Interface Block (3ph)/LConn1
  L1/LConn3 -- SSN Interface Block (3ph)/RConn3
  Subsystem/RConn1 -- L/LConn1
  Grid1/RConn1 -- Three-Phase Breaker/RConn1
  Grid1/RConn2 -- Three-Phase Breaker/RConn2
  Grid1/RConn3 -- Three-Phase Breaker/RConn3
  Three-Phase Breaker/LConn1 -- a/RConn1
  Three-Phase Breaker/LConn2 -- b/RConn1
  c/RConn1 -- Three-Phase Breaker/LConn3
  L2/RConn1 -- L2/RConn3 -- L2/RConn2

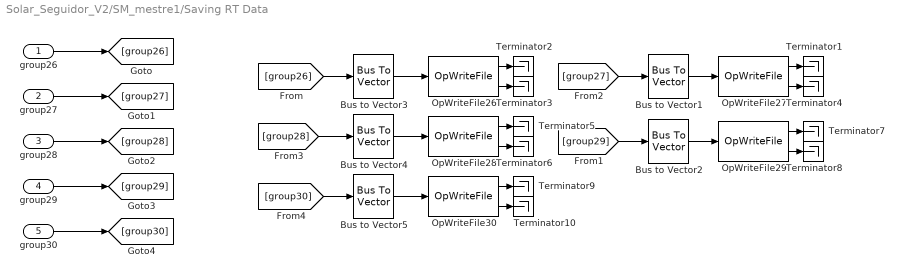
== system Solar_Seguidor_V2/SM_mestre1/Saving RT Data ==
  group26 : Inport
  group27 : Inport  Port=2
  group28 : Inport  Port=3
  group29 : Inport  Port=4
  group30 : Inport  Port=5
  Bus to Vector{1..5} (5 alike) : BusToVector
  OpWriteFile26 : rtlab/DataLogging/OpWriteFile  Static_File=on  varname=PV  Filename=PV_m.mat  rtpath='./'  nrtpath='.\'  Acq_Group=26  file_size=(nls26+1)*8*(ld26/Ts)*1.5  write_offline=on  Sim_Mode=off  Nb_Samples=ld26/Ts  Buffer_size=(ld26/Ts)*8*(1+nls26)
      settings: SourceProductName=RT-LAB  Decimation=Decimation26
  OpWriteFile27 : rtlab/DataLogging/OpWriteFile  Static_File=on  varname=Irra  Filename=Irradiance.mat  rtpath='./'  nrtpath='.\'  Acq_Group=27  file_size=(nls27+1)*8*(ld27/Ts)*1.5  write_offline=on  Sim_Mode=off  Nb_Samples=ld27/Ts  Buffer_size=(ld26/Ts)*8*(1+nls26)
      settings: SourceProductName=RT-LAB  Decimation=Decimation27
  OpWriteFile28 : rtlab/DataLogging/OpWriteFile  Static_File=on  varname=PV_mode  Filename=PV_mode.mat  rtpath='./'  nrtpath='.\'  Acq_Group=28  file_size=(nls28+1)*8*(ld28/Ts)*1.5  write_offline=on  Sim_Mode=off  Nb_Samples=ld28/Ts  Buffer_size=(ld28/Ts)*8*(1+nls28)
      settings: SourceProductName=RT-LAB  Decimation=Decimation28
  OpWriteFile29 : rtlab/DataLogging/OpWriteFile  Static_File=on  varname=BRK_PV  Filename=BRK_PV.mat  rtpath='./'  nrtpath='.\'  Acq_Group=29  file_size=(nls29+1)*8*(ld29/Ts)*1.5  write_offline=on  Sim_Mode=off  Nb_Samples=ld29/Ts  Buffer_size=(ld29/Ts)*8*(1+nls29)
      settings: SourceProductName=RT-LAB  Decimation=Decimation29
  OpWriteFile30 : rtlab/DataLogging/OpWriteFile  Static_File=on  varname=Iabc_grid  Filename=Iabc_grid.mat  rtpath='./'  nrtpath='.\'  Acq_Group=30  file_size=(nls30+1)*8*(ld30/Ts)*1.5  write_offline=on  Sim_Mode=off  Nb_Samples=ld30/Ts  Buffer_size=(ld30/Ts)*8*(1+nls30)
      settings: SourceProductName=RT-LAB  Decimation=Decimation30
  Terminator{1..10} (10 alike) : Terminator
  wires:
  OpWriteFile28/2 -> Terminator6/1
  OpWriteFile27/1 -> Terminator1/1
  OpWriteFile26/2 -> Terminator3/1
  OpWriteFile26/1 -> Terminator2/1
  OpWriteFile30/1 -> Terminator9/1
  OpWriteFile27/2 -> Terminator4/1
  OpWriteFile29/2 -> Terminator8/1
  OpWriteFile30/2 -> Terminator10/1
  OpWriteFile29/1 -> Terminator7/1
  OpWriteFile28/1 -> Terminator5/1
  group26/1 -> [group26]
  group27/1 -> [group27]
  group28/1 -> [group28]
  group29/1 -> [group29]
  group30/1 -> [group30]
  [group27] -> Bus to Vector1/1
  Bus to Vector1/1 -> OpWriteFile27/1
  [group29] -> Bus to Vector2/1
  Bus to Vector2/1 -> OpWriteFile29/1
  [group26] -> Bus to Vector3/1
  Bus to Vector3/1 -> OpWriteFile26/1
  [group28] -> Bus to Vector4/1
  Bus to Vector4/1 -> OpWriteFile28/1
  [group30] -> Bus to Vector5/1
  Bus to Vector5/1 -> OpWriteFile30/1

== system Solar_Seguidor_V2/SM_mestre1/eHS ==
  Ia_PV : Inport  PortDimensions=1
  Ib_PV : Inport  Port=2  PortDimensions=1
  Ic_PV : Inport  Port=3  PortDimensions=1
  Va_grid : Inport  Port=4  PortDimensions=1
  Vb_grid : Inport  Port=5  PortDimensions=1
  Vc_grid : Inport  Port=6  PortDimensions=1
  OpOutput_Ia_PV : rtlab/OpOutput  identifier_use=Ia_PV  identifier_hide=eHS/Ia_PV  nb_parents_identifier=1
      settings: SourceProductName=RT-LAB
  OpOutput_Ib_PV : rtlab/OpOutput  identifier_use=Ib_PV  identifier_hide=eHS/Ib_PV  nb_parents_identifier=1
      settings: SourceProductName=RT-LAB
  OpOutput_Ic_PV : rtlab/OpOutput  identifier_use=Ic_PV  identifier_hide=eHS/Ic_PV  nb_parents_identifier=1
      settings: SourceProductName=RT-LAB
  OpOutput_Va_grid : rtlab/OpOutput  identifier_use=Va_grid  identifier_hide=eHS/Va_grid  nb_parents_identifier=1
      settings: SourceProductName=RT-LAB
  OpOutput_Vb_grid : rtlab/OpOutput  identifier_use=Vb_grid  identifier_hide=eHS/Vb_grid  nb_parents_identifier=1
      settings: SourceProductName=RT-LAB
  OpOutput_Vc_grid : rtlab/OpOutput  identifier_use=Vc_grid  identifier_hide=eHS/Vc_grid  nb_parents_identifier=1
      settings: SourceProductName=RT-LAB
  OpOutput_parameter_set_id : rtlab/OpOutput  identifier_use=parameter_set_id  identifier_hide=eHS/parameter_set_id  nb_parents_identifier=1
      settings: SourceProductName=RT-LAB
  internal : Constant  Value=0
  internal_or_external : Constant  Value=0
  parameter_set_switch : Switch  Criteria=u2 > Threshold
  wires:
  Ia_PV/1 -> OpOutput_Ia_PV/1
  Ib_PV/1 -> OpOutput_Ib_PV/1
  Ic_PV/1 -> OpOutput_Ic_PV/1
  Va_grid/1 -> OpOutput_Va_grid/1
  Vb_grid/1 -> OpOutput_Vb_grid/1
  Vc_grid/1 -> OpOutput_Vc_grid/1
  internal_or_external/1 -> parameter_set_switch/2
  internal/1 -> parameter_set_switch/3
  parameter_set_switch/1 -> OpOutput_parameter_set_id/1

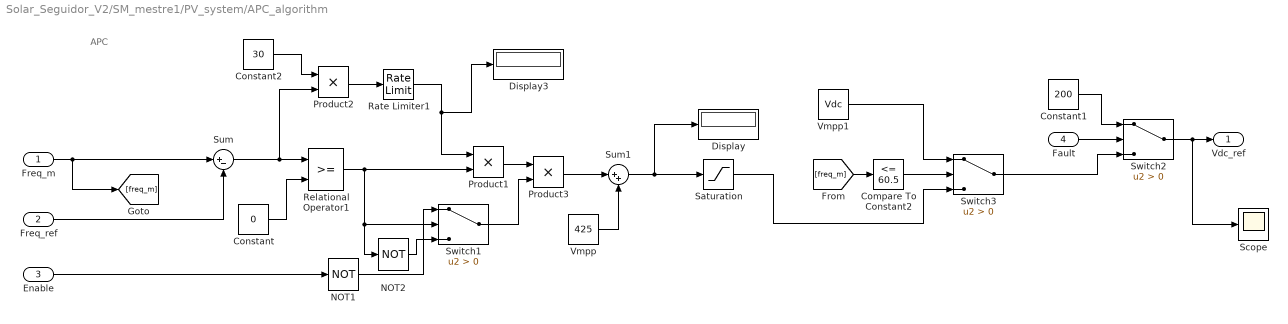
== system Solar_Seguidor_V2/SM_mestre1/PV_system/APC_algorithm ==
  note: APC
  Freq_m : Inport
  Freq_ref : Inport  Port=2
  Enable : Inport  Port=3
  Fault : Inport  Port=4
  Compare To Constant2 : simulink/Logic and Bit Operations/Compare To Constant  relop=<=  const=60.5  OutDataTypeStr=boolean
  Constant : Constant  Value=0
  Constant1 : Constant  Value=200
  Constant2 : Constant  Value=30
  Display : Display
  Display3 : Display
  NOT1 : Logic  Operator=NOT  IconShape=distinctive  AllPortsSameDT=off  OutDataTypeStr=boolean
  NOT2 : Logic  Operator=NOT  IconShape=distinctive  AllPortsSameDT=off  OutDataTypeStr=boolean
  Product1 : Product
  Product2 : Product
  Product3 : Product
  Rate Limiter1 : RateLimiter  RisingSlewLimit=200  FallingSlewLimit=-200  SampleTimeMode=inherited
  Relational Operator1 : RelationalOperator  OutDataTypeStr=boolean  RndMeth=Simplest
  Saturation : Saturate  UpperLimit=580  LowerLimit=0
  Scope : Scope
  Sum : Sum  Inputs=|+-
  Sum1 : Sum  Inputs=|++
  Switch1 : Switch  Criteria=u2 > Threshold
  Switch2 : Switch  Criteria=u2 > Threshold
  Switch3 : Switch  Criteria=u2 > Threshold
  Vmpp : Constant  Value=425
  Vmpp1 : Constant  Value=Vdc
  Vdc_ref : Outport
  wires:
  Product3/1 -> Sum1/1
  Sum1/1 -> Saturation/1, Display/1
  Product1/1 -> Product3/1
  Sum/1 -> Product2/2, Relational Operator1/1
  Switch1/1 -> Product3/2
  Relational Operator1/1 -> NOT2/1, Switch1/2, Product1/2
  NOT2/1 -> Switch1/3
  Constant2/1 -> Product2/1
  Product2/1 -> Rate Limiter1/1
  Rate Limiter1/1 -> Display3/1, Product1/1
  Enable/1 -> NOT1/1
  Vmpp/1 -> Sum1/2
  Constant/1 -> Relational Operator1/2
  Freq_m/1 -> Sum/1, [freq_m]
  NOT1/1 -> Switch1/1
  Freq_ref/1 -> Sum/2
  Switch2/1 -> Scope/1, Vdc_ref/1
  Fault/1 -> Switch2/2
  Constant1/1 -> Switch2/1
  [freq_m] -> Compare To Constant2/1
  Compare To Constant2/1 -> Switch3/2
  Saturation/1 -> Switch3/3
  Vmpp1/1 -> Switch3/1
  Switch3/1 -> Switch2/3

== system Solar_Seguidor_V2/SM_mestre1/PV_system/Subsystem ==
  Current Measurement : spsCurrentMeasurementLib/Current Measurement  PhasorSimulation=off  OutputType=Complex  PSBequivalent=0
  Current Measurement1 : spsCurrentMeasurementLib/Current Measurement  PhasorSimulation=off  OutputType=Complex  PSBequivalent=0
  Current Measurement2 : spsCurrentMeasurementLib/Current Measurement  PhasorSimulation=off  OutputType=Complex  PSBequivalent=0
  Mux : Mux  Inputs=3
  a : PMIOPort  Side=Left
  Va : PMIOPort  Port=2  Side=Right
  b : PMIOPort  Port=3  Side=Left
  Vb : PMIOPort  Port=4  Side=Right
  c : PMIOPort  Port=5  Side=Left
  Vc : PMIOPort  Port=6  Side=Right
  Iabc : Outport
  wires:
  Current Measurement1/1 -> Mux/2
  Mux/1 -> Iabc/1
  Current Measurement/1 -> Mux/1
  Current Measurement2/1 -> Mux/3
  connections:
  Current Measurement2/RConn1 -- Vc/RConn1
  Current Measurement1/RConn1 -- Vb/RConn1
  Current Measurement/LConn1 -- a/RConn1
  Current Measurement2/LConn1 -- c/RConn1
  Current Measurement/RConn1 -- Va/RConn1
  b/RConn1 -- Current Measurement1/LConn1

== system Solar_Seguidor_V2/SM_mestre1/PV_system/Subsystem1 ==
  Iabc : Inport
  In2 : Inport  Port=2
  Vdc : Inport  Port=3
  P_PV : Inport  Port=4
  Freq : Inport  Port=5
  Bus Creator : BusCreator  Inputs=6
  Gain5 : Gain  Gain=1/(Ibase*1.27)
  Gain6 : Gain  Gain=1/(Ibase*1.15)
  THD : Subsystem
  Out1 : Outport
  wires:
  Iabc/1 -> THD/1(Iabc), Gain5/1
  Bus Creator/1 -> Out1/1
  THD/1(THD_I) -> Bus Creator/1  "THD_Ia"
  Gain6/1 -> Bus Creator/3  "Iabc_grid_pu"
  Gain5/1 -> Bus Creator/2  "Iabc_PV_pu"
  Freq/1 -> Bus Creator/6
  Vdc/1 -> Bus Creator/4
  P_PV/1 -> Bus Creator/5
  In2/1 -> Gain6/1

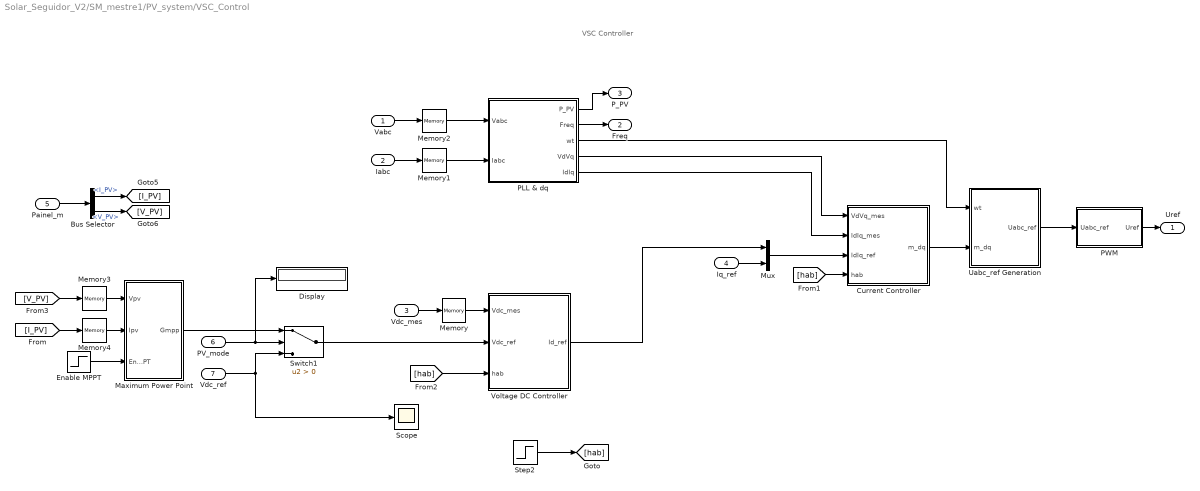
== system Solar_Seguidor_V2/SM_mestre1/PV_system/VSC_Control ==
  note: VSC Controller
  Vabc : Inport  PortDimensions=3
  Iabc : Inport  Port=2  PortDimensions=3
  Vdc_mes : Inport  Port=3
  Iq_ref : Inport  Port=4
  Painel_m : Inport  Port=5
  PV_mode : Inport  Port=6
  Vdc_ref : Inport  Port=7
  Bus Selector : BusSelector  OutputSignals=I_PV,V_PV
  Current Controller : Subsystem
  Display : Display
  Enable MPPT : Step  Time=0.4  SampleTime=0
  Maximum Power Point : Subsystem
  Memory{,1..4} (5 alike) : Memory
  Mux : Mux  Inputs=2
  PLL & dq : Subsystem
  PWM : Subsystem
  Scope : Scope
  Step2 : Step  Time=0  SampleTime=0
  Switch1 : Switch  Criteria=u2 > Threshold
  "Uabc_ref Generation " : Subsystem
  Voltage DC Controller : Subsystem
  Uref : Outport  VectorParamsAs1DForOutWhenUnconnected=off
  Freq : Outport  Port=2
  P_PV : Outport  Port=3
  wires:
  [hab] -> Current Controller/4(hab)
  "Uabc_ref Generation "/1(Uabc_ref) -> PWM/1(Uabc_ref)
  PLL & dq/2(Freq) -> Freq/1
  PLL & dq/3(wt) -> "Uabc_ref Generation "/1(wt)
  PLL & dq/5(IdIq) -> Current Controller/2(IdIq_mes)
  Mux/1 -> Current Controller/3(IdIq_ref)
  PLL & dq/4(VdVq) -> Current Controller/1(VdVq_mes)
  Iq_ref/1 -> Mux/2
  Current Controller/1(m_dq) -> "Uabc_ref Generation "/2(m_dq)
  Step2/1 -> [hab]
  [hab] -> Voltage DC Controller/3(hab)
  Vdc_mes/1 -> Memory/1
  PLL & dq/1(P_PV) -> P_PV/1
  Memory/1 -> Voltage DC Controller/1(Vdc_mes)
  Iabc/1 -> Memory1/1
  Memory1/1 -> PLL & dq/2(Iabc)
  Vabc/1 -> Memory2/1
  Memory2/1 -> PLL & dq/1(Vabc)
  Enable MPPT/1 -> Maximum Power Point/3(Enable_MPPT)
  Maximum Power Point/1(Gmpp) -> Switch1/1
  Voltage DC Controller/1(Id_ref) -> Mux/1
  Memory3/1 -> Maximum Power Point/1(Vpv)
  Memory4/1 -> Maximum Power Point/2(Ipv)
  PV_mode/1 -> Switch1/2, Display/1
  Vdc_ref/1 -> Switch1/3, Scope/1
  Switch1/1 -> Voltage DC Controller/2(Vdc_ref)
  Bus Selector/2 -> [V_PV]  "<V_PV>"
  Bus Selector/1 -> [I_PV]  "<I_PV>"
  Painel_m/1 -> Bus Selector/1
  [I_PV] -> Memory4/1
  [V_PV] -> Memory3/1
  PWM/1(Uref) -> Uref/1

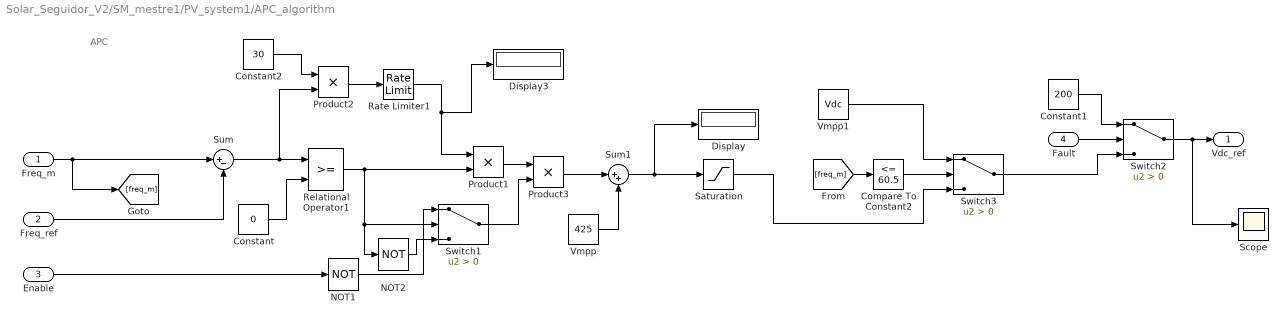
== system Solar_Seguidor_V2/SM_mestre1/PV_system1/APC_algorithm ==
  note: APC
  Freq_m : Inport
  Freq_ref : Inport  Port=2
  Enable : Inport  Port=3
  Fault : Inport  Port=4
  Compare To Constant2 : simulink/Logic and Bit Operations/Compare To Constant  relop=<=  const=60.5  OutDataTypeStr=boolean
  Constant : Constant  Value=0
  Constant1 : Constant  Value=200
  Constant2 : Constant  Value=30
  Display : Display
  Display3 : Display
  NOT1 : Logic  Operator=NOT  IconShape=distinctive  AllPortsSameDT=off  OutDataTypeStr=boolean
  NOT2 : Logic  Operator=NOT  IconShape=distinctive  AllPortsSameDT=off  OutDataTypeStr=boolean
  Product1 : Product
  Product2 : Product
  Product3 : Product
  Rate Limiter1 : RateLimiter  RisingSlewLimit=200  FallingSlewLimit=-200  SampleTimeMode=inherited
  Relational Operator1 : RelationalOperator  OutDataTypeStr=boolean  RndMeth=Simplest
  Saturation : Saturate  UpperLimit=580  LowerLimit=0
  Scope : Scope
  Sum : Sum  Inputs=|+-
  Sum1 : Sum  Inputs=|++
  Switch1 : Switch  Criteria=u2 > Threshold
  Switch2 : Switch  Criteria=u2 > Threshold
  Switch3 : Switch  Criteria=u2 > Threshold
  Vmpp : Constant  Value=425
  Vmpp1 : Constant  Value=Vdc
  Vdc_ref : Outport
  wires:
  Switch3/1 -> Switch2/3
  Vmpp1/1 -> Switch3/1
  Saturation/1 -> Switch3/3
  Compare To Constant2/1 -> Switch3/2
  [freq_m] -> Compare To Constant2/1
  Constant1/1 -> Switch2/1
  Fault/1 -> Switch2/2
  Switch2/1 -> Vdc_ref/1, Scope/1
  Freq_ref/1 -> Sum/2
  NOT1/1 -> Switch1/1
  Freq_m/1 -> [freq_m], Sum/1
  Constant/1 -> Relational Operator1/2
  Vmpp/1 -> Sum1/2
  Enable/1 -> NOT1/1
  Rate Limiter1/1 -> Product1/1, Display3/1
  Product2/1 -> Rate Limiter1/1
  Constant2/1 -> Product2/1
  NOT2/1 -> Switch1/3
  Relational Operator1/1 -> Product1/2, Switch1/2, NOT2/1
  Switch1/1 -> Product3/2
  Sum/1 -> Relational Operator1/1, Product2/2
  Product1/1 -> Product3/1
  Sum1/1 -> Display/1, Saturation/1
  Product3/1 -> Sum1/1

== system Solar_Seguidor_V2/SM_mestre1/PV_system1/Subsystem ==
  Current Measurement : spsCurrentMeasurementLib/Current Measurement  PhasorSimulation=off  OutputType=Complex  PSBequivalent=0
  Current Measurement1 : spsCurrentMeasurementLib/Current Measurement  PhasorSimulation=off  OutputType=Complex  PSBequivalent=0
  Current Measurement2 : spsCurrentMeasurementLib/Current Measurement  PhasorSimulation=off  OutputType=Complex  PSBequivalent=0
  Mux : Mux  Inputs=3
  a : PMIOPort  Side=Left
  Va : PMIOPort  Port=2  Side=Right
  b : PMIOPort  Port=3  Side=Left
  Vb : PMIOPort  Port=4  Side=Right
  c : PMIOPort  Port=5  Side=Left
  Vc : PMIOPort  Port=6  Side=Right
  Iabc : Outport
  wires:
  Current Measurement2/1 -> Mux/3
  Current Measurement/1 -> Mux/1
  Mux/1 -> Iabc/1
  Current Measurement1/1 -> Mux/2
  connections:
  b/RConn1 -- Current Measurement1/LConn1
  Current Measurement/RConn1 -- Va/RConn1
  Current Measurement2/LConn1 -- c/RConn1
  Current Measurement/LConn1 -- a/RConn1
  Current Measurement1/RConn1 -- Vb/RConn1
  Current Measurement2/RConn1 -- Vc/RConn1

== system Solar_Seguidor_V2/SM_mestre1/PV_system1/Subsystem1 ==
  Iabc : Inport
  In2 : Inport  Port=2
  Vdc : Inport  Port=3
  P_PV : Inport  Port=4
  Freq : Inport  Port=5
  Bus Creator : BusCreator  Inputs=6
  Gain5 : Gain  Gain=1/(Ibase*1.27)
  Gain6 : Gain  Gain=1/(Ibase*1.15)
  THD : Subsystem
  Out1 : Outport
  wires:
  In2/1 -> Gain6/1
  P_PV/1 -> Bus Creator/5
  Vdc/1 -> Bus Creator/4
  Freq/1 -> Bus Creator/6
  Gain5/1 -> Bus Creator/2  "Iabc_PV_pu"
  Gain6/1 -> Bus Creator/3  "Iabc_grid_pu"
  THD/1(THD_I) -> Bus Creator/1  "THD_Ia"
  Bus Creator/1 -> Out1/1
  Iabc/1 -> Gain5/1, THD/1(Iabc)

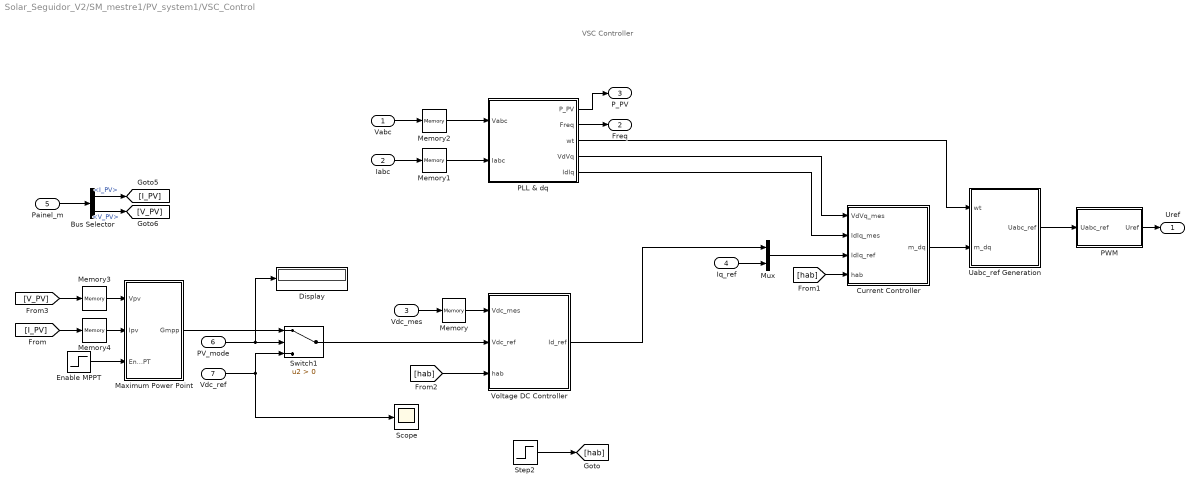
== system Solar_Seguidor_V2/SM_mestre1/PV_system1/VSC_Control ==
  note: VSC Controller
  Vabc : Inport  PortDimensions=3
  Iabc : Inport  Port=2  PortDimensions=3
  Vdc_mes : Inport  Port=3
  Iq_ref : Inport  Port=4
  Painel_m : Inport  Port=5
  PV_mode : Inport  Port=6
  Vdc_ref : Inport  Port=7
  Bus Selector : BusSelector  OutputSignals=I_PV,V_PV
  Current Controller : Subsystem
  Display : Display
  Enable MPPT : Step  Time=0.4  SampleTime=0
  Maximum Power Point : Subsystem
  Memory{,1..4} (5 alike) : Memory
  Mux : Mux  Inputs=2
  PLL & dq : Subsystem
  PWM : Subsystem
  Scope : Scope
  Step2 : Step  Time=0  SampleTime=0
  Switch1 : Switch  Criteria=u2 > Threshold
  "Uabc_ref Generation " : Subsystem
  Voltage DC Controller : Subsystem
  Uref : Outport  VectorParamsAs1DForOutWhenUnconnected=off
  Freq : Outport  Port=2
  P_PV : Outport  Port=3
  wires:
  PWM/1(Uref) -> Uref/1
  [V_PV] -> Memory3/1
  [I_PV] -> Memory4/1
  Painel_m/1 -> Bus Selector/1
  Bus Selector/1 -> [I_PV]  "<I_PV>"
  Bus Selector/2 -> [V_PV]  "<V_PV>"
  Switch1/1 -> Voltage DC Controller/2(Vdc_ref)
  Vdc_ref/1 -> Scope/1, Switch1/3
  PV_mode/1 -> Display/1, Switch1/2
  Memory4/1 -> Maximum Power Point/2(Ipv)
  Memory3/1 -> Maximum Power Point/1(Vpv)
  Voltage DC Controller/1(Id_ref) -> Mux/1
  Maximum Power Point/1(Gmpp) -> Switch1/1
  Enable MPPT/1 -> Maximum Power Point/3(Enable_MPPT)
  Memory2/1 -> PLL & dq/1(Vabc)
  Vabc/1 -> Memory2/1
  Memory1/1 -> PLL & dq/2(Iabc)
  Iabc/1 -> Memory1/1
  Memory/1 -> Voltage DC Controller/1(Vdc_mes)
  PLL & dq/1(P_PV) -> P_PV/1
  Vdc_mes/1 -> Memory/1
  [hab] -> Voltage DC Controller/3(hab)
  Step2/1 -> [hab]
  Current Controller/1(m_dq) -> "Uabc_ref Generation "/2(m_dq)
  Iq_ref/1 -> Mux/2
  PLL & dq/4(VdVq) -> Current Controller/1(VdVq_mes)
  Mux/1 -> Current Controller/3(IdIq_ref)
  PLL & dq/5(IdIq) -> Current Controller/2(IdIq_mes)
  PLL & dq/3(wt) -> "Uabc_ref Generation "/1(wt)
  PLL & dq/2(Freq) -> Freq/1
  "Uabc_ref Generation "/1(Uabc_ref) -> PWM/1(Uabc_ref)
  [hab] -> Current Controller/4(hab)

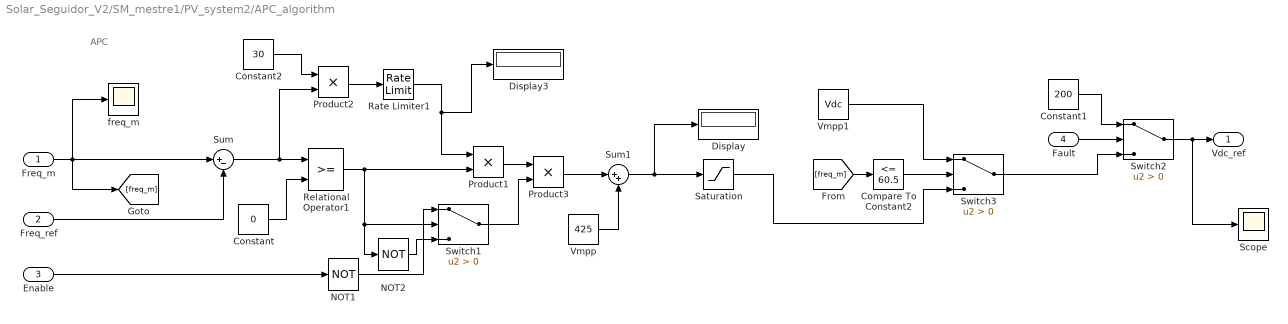
== system Solar_Seguidor_V2/SM_mestre1/PV_system2/APC_algorithm ==
  note: APC
  Freq_m : Inport
  Freq_ref : Inport  Port=2
  Enable : Inport  Port=3
  Fault : Inport  Port=4
  Compare To Constant2 : simulink/Logic and Bit Operations/Compare To Constant  relop=<=  const=60.5  OutDataTypeStr=boolean
  Constant : Constant  Value=0
  Constant1 : Constant  Value=200
  Constant2 : Constant  Value=30
  Display : Display
  Display3 : Display
  NOT1 : Logic  Operator=NOT  IconShape=distinctive  AllPortsSameDT=off  OutDataTypeStr=boolean
  NOT2 : Logic  Operator=NOT  IconShape=distinctive  AllPortsSameDT=off  OutDataTypeStr=boolean
  Product1 : Product
  Product2 : Product
  Product3 : Product
  Rate Limiter1 : RateLimiter  RisingSlewLimit=200  FallingSlewLimit=-200  SampleTimeMode=inherited
  Relational Operator1 : RelationalOperator  OutDataTypeStr=boolean  RndMeth=Simplest
  Saturation : Saturate  UpperLimit=580  LowerLimit=0
  Scope : Scope
  Sum : Sum  Inputs=|+-
  Sum1 : Sum  Inputs=|++
  Switch1 : Switch  Criteria=u2 > Threshold
  Switch2 : Switch  Criteria=u2 > Threshold
  Switch3 : Switch  Criteria=u2 > Threshold
  Vmpp : Constant  Value=425
  Vmpp1 : Constant  Value=Vdc
  freq_m : Scope
  Vdc_ref : Outport
  wires:
  Switch3/1 -> Switch2/3
  Vmpp1/1 -> Switch3/1
  Saturation/1 -> Switch3/3
  Compare To Constant2/1 -> Switch3/2
  [freq_m] -> Compare To Constant2/1
  Constant1/1 -> Switch2/1
  Fault/1 -> Switch2/2
  Switch2/1 -> Vdc_ref/1, Scope/1
  Freq_ref/1 -> Sum/2
  NOT1/1 -> Switch1/1
  Freq_m/1 -> [freq_m], Sum/1, freq_m/1
  Constant/1 -> Relational Operator1/2
  Vmpp/1 -> Sum1/2
  Enable/1 -> NOT1/1
  Rate Limiter1/1 -> Product1/1, Display3/1
  Product2/1 -> Rate Limiter1/1
  Constant2/1 -> Product2/1
  NOT2/1 -> Switch1/3
  Relational Operator1/1 -> Product1/2, Switch1/2, NOT2/1
  Switch1/1 -> Product3/2
  Sum/1 -> Relational Operator1/1, Product2/2
  Product1/1 -> Product3/1
  Sum1/1 -> Display/1, Saturation/1
  Product3/1 -> Sum1/1

== system Solar_Seguidor_V2/SM_mestre1/PV_system2/Subsystem ==
  Current Measurement : spsCurrentMeasurementLib/Current Measurement  PhasorSimulation=off  OutputType=Complex  PSBequivalent=0
  Current Measurement1 : spsCurrentMeasurementLib/Current Measurement  PhasorSimulation=off  OutputType=Complex  PSBequivalent=0
  Current Measurement2 : spsCurrentMeasurementLib/Current Measurement  PhasorSimulation=off  OutputType=Complex  PSBequivalent=0
  Mux : Mux  Inputs=3
  a : PMIOPort  Side=Left
  Va : PMIOPort  Port=2  Side=Right
  b : PMIOPort  Port=3  Side=Left
  Vb : PMIOPort  Port=4  Side=Right
  c : PMIOPort  Port=5  Side=Left
  Vc : PMIOPort  Port=6  Side=Right
  Iabc : Outport
  wires:
  Current Measurement2/1 -> Mux/3
  Current Measurement/1 -> Mux/1
  Mux/1 -> Iabc/1
  Current Measurement1/1 -> Mux/2
  connections:
  b/RConn1 -- Current Measurement1/LConn1
  Current Measurement/RConn1 -- Va/RConn1
  Current Measurement2/LConn1 -- c/RConn1
  Current Measurement/LConn1 -- a/RConn1
  Current Measurement1/RConn1 -- Vb/RConn1
  Current Measurement2/RConn1 -- Vc/RConn1

== system Solar_Seguidor_V2/SM_mestre1/PV_system2/Subsystem1 ==
  Iabc : Inport
  In2 : Inport  Port=2
  Vdc : Inport  Port=3
  P_PV : Inport  Port=4
  Freq : Inport  Port=5
  Bus Creator : BusCreator  Inputs=6
  Gain5 : Gain  Gain=1/(Ibase*1.27)
  Gain6 : Gain  Gain=1/(Ibase*1.15)
  THD : Subsystem
  PV_m : Outport
  wires:
  In2/1 -> Gain6/1
  P_PV/1 -> Bus Creator/5
  Vdc/1 -> Bus Creator/4
  Freq/1 -> Bus Creator/6
  Gain5/1 -> Bus Creator/2  "Iabc_PV_pu"
  Gain6/1 -> Bus Creator/3  "Iabc_grid_pu"
  THD/1(THD_I) -> Bus Creator/1  "THD_Ia"
  Bus Creator/1 -> PV_m/1
  Iabc/1 -> Gain5/1, THD/1(Iabc)

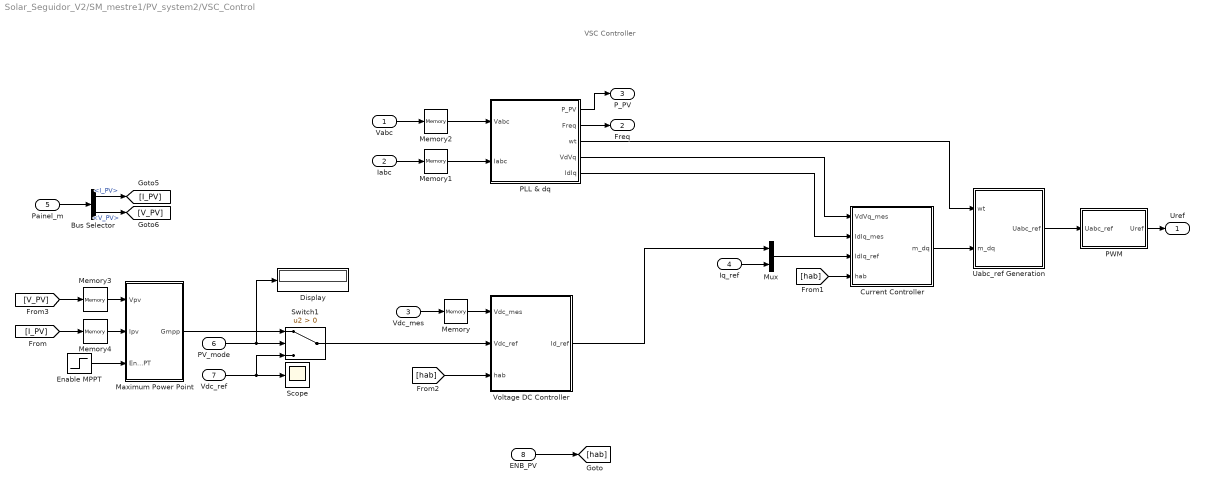
== system Solar_Seguidor_V2/SM_mestre1/PV_system2/VSC_Control ==
  note: VSC Controller
  Vabc : Inport  PortDimensions=3
  Iabc : Inport  Port=2  PortDimensions=3
  Vdc_mes : Inport  Port=3
  Iq_ref : Inport  Port=4
  Painel_m : Inport  Port=5
  PV_mode : Inport  Port=6
  Vdc_ref : Inport  Port=7
  ENB_PV : Inport  Port=8
  Bus Selector : BusSelector  OutputSignals=I_PV,V_PV
  Current Controller : Subsystem
  Display : Display
  Enable MPPT : Step  Time=0  SampleTime=0
  Maximum Power Point : Subsystem
  Memory{,1..4} (5 alike) : Memory
  Mux : Mux  Inputs=2
  PLL & dq : Subsystem
  PWM : Subsystem
  Scope : Scope
  Switch1 : Switch  Criteria=u2 > Threshold
  "Uabc_ref Generation " : Subsystem
  Voltage DC Controller : Subsystem
  Uref : Outport  VectorParamsAs1DForOutWhenUnconnected=off
  Freq : Outport  Port=2
  P_PV : Outport  Port=3
  wires:
  PWM/1(Uref) -> Uref/1
  [V_PV] -> Memory3/1
  [I_PV] -> Memory4/1
  Painel_m/1 -> Bus Selector/1
  Bus Selector/1 -> [I_PV]  "<I_PV>"
  Bus Selector/2 -> [V_PV]  "<V_PV>"
  Switch1/1 -> Voltage DC Controller/2(Vdc_ref)
  Vdc_ref/1 -> Scope/1, Switch1/3
  PV_mode/1 -> Display/1, Switch1/2
  Memory4/1 -> Maximum Power Point/2(Ipv)
  Memory3/1 -> Maximum Power Point/1(Vpv)
  Voltage DC Controller/1(Id_ref) -> Mux/1
  Maximum Power Point/1(Gmpp) -> Switch1/1
  Enable MPPT/1 -> Maximum Power Point/3(Enable_MPPT)
  Memory2/1 -> PLL & dq/1(Vabc)
  Vabc/1 -> Memory2/1
  Memory1/1 -> PLL & dq/2(Iabc)
  Iabc/1 -> Memory1/1
  Memory/1 -> Voltage DC Controller/1(Vdc_mes)
  PLL & dq/1(P_PV) -> P_PV/1
  Vdc_mes/1 -> Memory/1
  [hab] -> Voltage DC Controller/3(hab)
  ENB_PV/1 -> [hab]
  Current Controller/1(m_dq) -> "Uabc_ref Generation "/2(m_dq)
  Iq_ref/1 -> Mux/2
  PLL & dq/4(VdVq) -> Current Controller/1(VdVq_mes)
  Mux/1 -> Current Controller/3(IdIq_ref)
  PLL & dq/5(IdIq) -> Current Controller/2(IdIq_mes)
  PLL & dq/3(wt) -> "Uabc_ref Generation "/1(wt)
  PLL & dq/2(Freq) -> Freq/1
  "Uabc_ref Generation "/1(Uabc_ref) -> PWM/1(Uabc_ref)
  [hab] -> Current Controller/4(hab)
